simulink model "sampleModel2049_1_sub_sub"  (R2023a)
settings: Solver=VariableStepAuto  StartTime=0.0  StopTime=10.0  RelTol=1e-3
libraries: hdlsllib x3, simulink x2
settings Model: Creator=user1  LastModifiedBy=user1

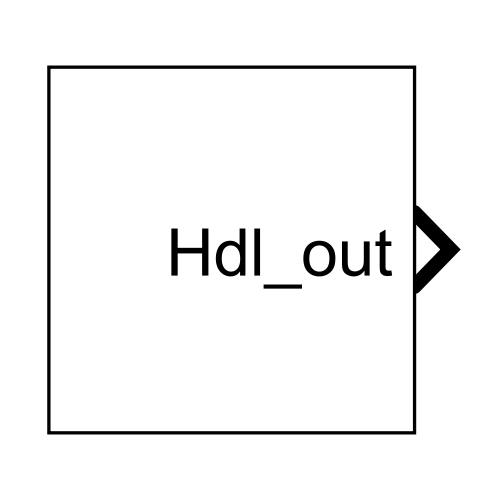
[thumbnail: Simulink's stored preview of the top-level diagram]
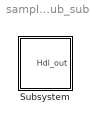
== system sampleModel2049_1_sub_sub ==
  Subsystem : Subsystem

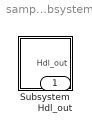
== system sampleModel2049_1_sub_sub/Subsystem ==
  Subsystem : Subsystem
  Hdl_out : Outport  OutDataTypeStr=uint8

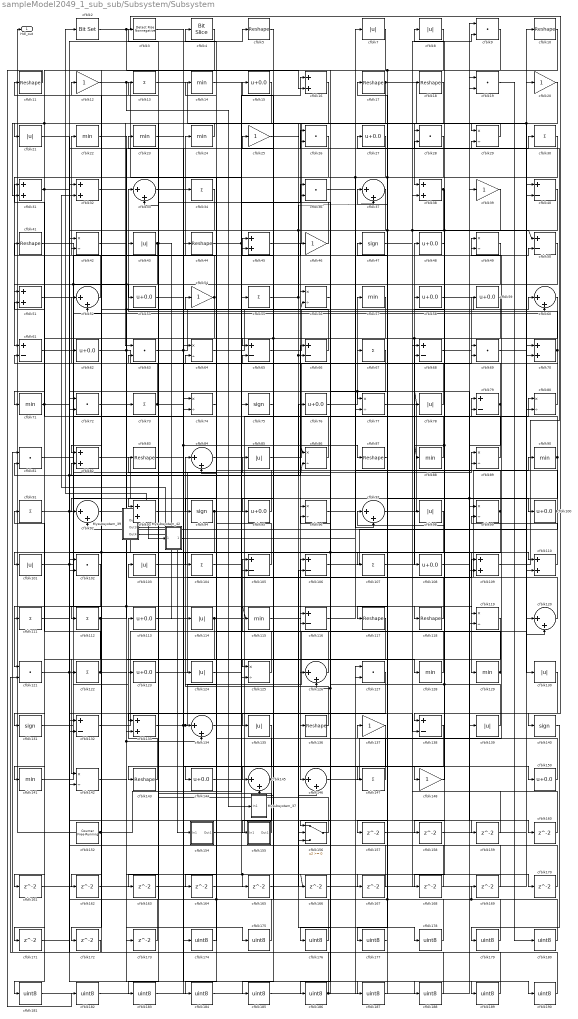
== system sampleModel2049_1_sub_sub/Subsystem/Subsystem ==
  Mysubsystem_37 : Subsystem  TreatAsAtomicUnit=on  RTWFcnName=Mysubsystem_37
      settings: RTWFcnNameOpts=User specified  RTWFileNameOpts=Use function name
  Mysubsystem_39 : Subsystem  TreatAsAtomicUnit=on  RTWFcnName=Mysubsystem_39
      settings: RTWFcnNameOpts=User specified  RTWFileNameOpts=Use function name
  Mysubsystem_42 : Subsystem  TreatAsAtomicUnit=on  RTWFcnName=Mysubsystem_42
      settings: RTWFcnNameOpts=User specified  RTWFileNameOpts=Use function name
  cfblk{5,10..11,17..18,41,44,83,87,117..118,136,143} (13 alike) : Reshape
  cfblk{15,27,48,53,58..59,62,76,95,100,108,113,123,144,150} (15 alike) : Bias  Bias=0.0  SaturateOnIntegerOverflow=off
  cfblk{7..8,21,43,78,85,98,101,103,114,124,130,135,139} (14 alike) : Abs  OutDataTypeStr=uint8  SaturateOnIntegerOverflow=off
  cfblk{9,19,26,28,36,63,69,72,81,102,121,127} (12 alike) : DotProduct  OutDataTypeStr=uint8
  cfblk{13,30,34,55,67,73,91,104,107,111..112,122,147} (13 alike) : Sum  Inputs=+  OutDataTypeStr=uint8
  cfblk{40,50,61,65..66,68,79,105..106,116,132,138} (12 alike) : Sum  Inputs=+-  OutDataTypeStr=uint8
  cfblk{16,31..32,38,45,51,70,82,93,109..110,133} (12 alike) : Sum  OutDataTypeStr=uint8
  cfblk{14,22..24,57,71,88,90,115,128..129,141} (12 alike) : MinMax  OutDataTypeStr=uint8
  cfblk{29,42,49,56,64,74,77,80,86,89,96,99,119,125,142} (15 alike) : Product  Inputs=*/  OutDataTypeStr=uint8  RndMeth=Zero  SaturateOnIntegerOverflow=on
  cfblk{12,20,25,39,46,54,137,148} (8 alike) : Gain  OutDataTypeStr=uint8
  cfblk{33,37,52,60,84,92,97,120,126,134,145..146} (12 alike) : Sum  Inputs=|++  OutDataTypeStr=uint8
  cfblk{47,75,94,131,140} (5 alike) : Signum
  cfblk152 : hdlsllib/Sources/Counter Free-Running  NumBits=16  tsamp=-1
  cfblk154 : Subsystem
      settings: LibrarySourceBlock=|
      | hdlsllib/Ports &
      | Subsystems/Subsystem
  cfblk155 : Subsystem
      settings: LibrarySourceBlock=|
      | hdlsllib/Ports &
      | Subsystems/Subsystem
  cfblk156 : Switch  OutDataTypeStr=uint8  SaturateOnIntegerOverflow=off  InputSameDT=off
  cfblk{157..173} (17 alike) : Delay  SampleTime=1
  cfblk{174..190} (17 alike) : DataTypeConversion  OutDataTypeStr=uint8  SaturateOnIntegerOverflow=off  RndMeth=Floor
  cfblk2 : simulink/Logic and Bit Operations/Bit Set  iBit=0
      settings: LibrarySourceBlock=|
      | hdlsllib/Logic and Bit
      | Operations/Bit Set
  cfblk3 : hdlsllib/Logic and Bit Operations/Detect Rise Nonnegative  vinit=0  OutDataTypeStr=uint8
  cfblk4 : hdlsllib/Logic and Bit Operations/Bit Slice  lidx=7  ridx=0
  Hdl_out : Outport  OutDataTypeStr=uint8
  wires:
  Mysubsystem_42/1(Out1) -> cfblk7/1
  Mysubsystem_39/2(Out2) -> Mysubsystem_42/1(In1)
  Mysubsystem_39/4(Out4) -> cfblk154/1(In1)
  Mysubsystem_39/3(Out3) -> cfblk32/2
  Mysubsystem_39/1(Y) -> cfblk2/1
  cfblk190/1 -> cfblk42/2
  cfblk189/1 -> cfblk42/1
  cfblk83/1 -> cfblk189/1
  cfblk188/1 -> cfblk81/1
  cfblk42/1 -> cfblk188/1
  cfblk187/1 -> cfblk137/1
  cfblk186/1 -> cfblk126/2, cfblk36/2, cfblk32/1
  cfblk185/1 -> cfblk127/2
  cfblk5/1 -> cfblk185/1
  cfblk184/1 -> cfblk127/1
  cfblk49/1 -> cfblk184/1
  cfblk183/1 -> cfblk44/1
  cfblk127/1 -> cfblk183/1
  cfblk182/1 -> cfblk19/2
  cfblk11/1 -> cfblk182/1
  cfblk181/1 -> cfblk19/1
  cfblk180/1 -> cfblk145/2, cfblk17/1, cfblk169/1
  cfblk179/1 -> cfblk25/1
  cfblk140/1 -> cfblk179/1
  cfblk178/1 -> cfblk43/1, cfblk54/1
  cfblk177/1 -> cfblk67/1
  cfblk176/1 -> cfblk72/1
  cfblk67/1 -> cfblk176/1
  cfblk175/1 -> cfblk3/1
  cfblk174/1 -> cfblk124/1
  cfblk3/1 -> cfblk174/1
  cfblk173/1 -> cfblk52/2
  cfblk22/1 -> cfblk173/1
  cfblk172/1 -> cfblk121/2
  cfblk34/1 -> cfblk172/1
  cfblk171/1 -> cfblk132/1
  cfblk170/1 -> cfblk33/2
  cfblk14/1 -> cfblk170/1
  cfblk169/1 -> cfblk63/2
  cfblk168/1 -> cfblk102/1
  cfblk130/1 -> cfblk168/1
  cfblk167/1 -> cfblk105/2
  cfblk166/1 -> cfblk120/2
  cfblk165/1 -> cfblk106/2
  cfblk164/1 -> cfblk146/2
  cfblk163/1 -> cfblk64/1
  cfblk60/1 -> cfblk163/1
  cfblk162/1 -> cfblk38/2
  cfblk37/1 -> cfblk162/1
  cfblk161/1 -> cfblk74/1
  cfblk57/1 -> cfblk161/1
  cfblk160/1 -> cfblk68/1
  cfblk108/1 -> cfblk160/1
  cfblk159/1 -> cfblk99/1
  cfblk158/1 -> cfblk70/1
  cfblk157/1 -> cfblk40/1
  cfblk87/1 -> cfblk157/1
  cfblk104/1 -> cfblk16/1
  cfblk64/1 -> cfblk40/2
  cfblk4/1 -> cfblk21/1
  cfblk16/1 -> cfblk156/2, cfblk66/2
  cfblk120/1 -> cfblk13/1
  cfblk98/1 -> cfblk122/1, cfblk171/1
  cfblk77/1 -> cfblk79/2
  cfblk9/1 -> cfblk156/1
  cfblk56/1 -> cfblk126/1
  cfblk122/1 -> cfblk91/1, cfblk175/1
  cfblk103/1 -> cfblk76/1
  cfblk156/1 -> cfblk23/1
  cfblk94/1 -> cfblk50/2, cfblk111/1
  cfblk10/1 -> cfblk82/1, cfblk177/1
  cfblk142/1 -> cfblk165/1, cfblk166/1
  cfblk105/1 -> cfblk64/2
  cfblk106/1 -> cfblk20/1
  cfblk12/1 -> Mysubsystem_37/1(In1), cfblk55/1
  cfblk73/1 -> cfblk86/1, cfblk125/2, cfblk31/1
  cfblk93/1 -> cfblk66/1
  cfblk69/1 -> cfblk130/1
  cfblk80/1 -> cfblk28/2
  cfblk65/1 -> cfblk9/1
  cfblk72/1 -> cfblk134/2, cfblk187/1
  cfblk55/1 -> cfblk118/1, cfblk37/2
  cfblk85/1 -> cfblk69/1
  cfblk131/1 -> cfblk123/1
  cfblk144/1 -> cfblk106/1
  cfblk68/1 -> cfblk59/1
  cfblk113/1 -> cfblk109/1
  cfblk19/1 -> cfblk180/1
  cfblk112/1 -> cfblk29/2, cfblk115/1, cfblk142/2
  cfblk134/1 -> cfblk75/1
  cfblk63/1 -> cfblk10/1, cfblk110/2
  cfblk119/1 -> cfblk142/1
  cfblk88/1 -> cfblk51/2
  cfblk129/1 -> cfblk96/2, cfblk49/2
  cfblk62/1 -> cfblk56/2, cfblk26/1, cfblk69/2
  cfblk118/1 -> cfblk37/1
  cfblk48/1 -> cfblk138/1
  cfblk132/1 -> cfblk18/1
  cfblk116/1 -> cfblk89/2
  cfblk31/1 -> cfblk77/1, cfblk78/1, cfblk51/1
  cfblk110/1 -> cfblk99/2
  cfblk90/1 -> cfblk107/1, cfblk109/2, cfblk68/2
  cfblk44/1 -> cfblk36/1, cfblk167/1
  cfblk20/1 -> cfblk70/2, cfblk65/1
  cfblk79/1 -> cfblk8/1, cfblk119/2
  cfblk36/1 -> cfblk97/2
  cfblk117/1 -> cfblk131/1
  cfblk95/1 -> cfblk41/1
  cfblk115/1 -> cfblk116/2
  cfblk32/1 -> cfblk125/1
  cfblk53/1 -> cfblk150/1
  cfblk21/1 -> cfblk110/1
  cfblk111/1 -> cfblk119/1
  cfblk75/1 -> cfblk95/1
  cfblk138/1 -> cfblk143/1
  cfblk7/1 -> cfblk112/1
  cfblk17/1 -> cfblk120/1, cfblk53/1
  cfblk50/1 -> cfblk101/1
  cfblk147/1 -> cfblk81/2
  cfblk43/1 -> cfblk72/2, cfblk133/2, cfblk114/1, cfblk93/1
  cfblk124/1 -> cfblk45/2
  cfblk27/1 -> cfblk71/1
  cfblk121/1 -> cfblk86/2, cfblk26/2, cfblk159/1
  cfblk29/1 -> cfblk28/1
  cfblk126/1 -> cfblk84/2
  cfblk78/1 -> cfblk52/1
  cfblk89/1 -> cfblk47/1
  cfblk30/1 -> cfblk92/1, cfblk147/1
  cfblk25/1 -> cfblk178/1
  cfblk46/1 -> cfblk12/1
  cfblk91/1 -> cfblk34/1, cfblk138/2
  cfblk86/1 -> cfblk15/1
  cfblk102/1 -> cfblk121/1
  cfblk133/1 -> cfblk80/2, cfblk134/1, cfblk30/1
  cfblk152/1 -> cfblk49/1, Hdl_out/1
  cfblk145/1 -> cfblk155/1(In1), cfblk61/2
  cfblk28/1 -> cfblk77/2, cfblk164/1
  cfblk47/1 -> cfblk50/1, cfblk9/2
  cfblk84/1 -> cfblk87/1
  cfblk99/1 -> cfblk136/1, cfblk132/2, cfblk62/1
  cfblk76/1 -> cfblk57/1
  cfblk135/1 -> cfblk145/1
  cfblk92/1 -> cfblk129/1
  cfblk150/1 -> cfblk83/1
  cfblk100/1 -> cfblk14/1, cfblk92/2
  cfblk8/1 -> cfblk56/1
  cfblk71/1 -> cfblk5/1, cfblk141/1
  cfblk123/1 -> cfblk89/1
  cfblk38/1 -> cfblk102/2, cfblk158/1
  cfblk148/1 -> cfblk58/1
  cfblk18/1 -> cfblk38/1
  cfblk82/1 -> cfblk96/1
  cfblk40/1 -> cfblk88/1, cfblk148/1, cfblk144/1, cfblk156/3
  cfblk96/1 -> cfblk98/1
  cfblk59/1 -> cfblk135/1, cfblk94/1, cfblk108/1
  cfblk137/1 -> cfblk186/1
  cfblk128/1 -> cfblk45/1
  cfblk136/1 -> cfblk84/1
  cfblk66/1 -> cfblk11/1
  cfblk52/1 -> cfblk22/1
  cfblk114/1 -> cfblk39/1, cfblk133/1
  cfblk39/1 -> cfblk117/1, cfblk104/1
  cfblk33/1 -> cfblk74/2
  cfblk155/1(Out1) -> cfblk103/1
  cfblk41/1 -> cfblk139/1, cfblk73/1
  cfblk141/1 -> cfblk85/1
  cfblk61/1 -> cfblk116/1
  cfblk51/1 -> cfblk100/1
  cfblk2/1 -> cfblk140/1, cfblk16/2
  cfblk125/1 -> cfblk105/1
  cfblk81/1 -> cfblk60/2
  cfblk143/1 -> cfblk113/1
  cfblk101/1 -> cfblk46/1, cfblk190/1
  cfblk13/1 -> cfblk146/1
  cfblk26/1 -> cfblk61/1
  cfblk97/1 -> cfblk79/1
  cfblk45/1 -> cfblk29/1
  cfblk15/1 -> cfblk31/2, cfblk181/1
  cfblk107/1 -> cfblk48/1
  cfblk74/1 -> cfblk4/1
  cfblk58/1 -> cfblk60/1
  cfblk24/1 -> cfblk63/1
  cfblk146/1 -> cfblk90/1
  cfblk139/1 -> cfblk97/1, cfblk82/2
  cfblk109/1 -> cfblk27/1
  cfblk23/1 -> cfblk128/1
  cfblk70/1 -> cfblk33/1, cfblk65/2
  cfblk54/1 -> cfblk24/1, cfblk93/2
  cfblk154/1(Out1) -> cfblk80/1

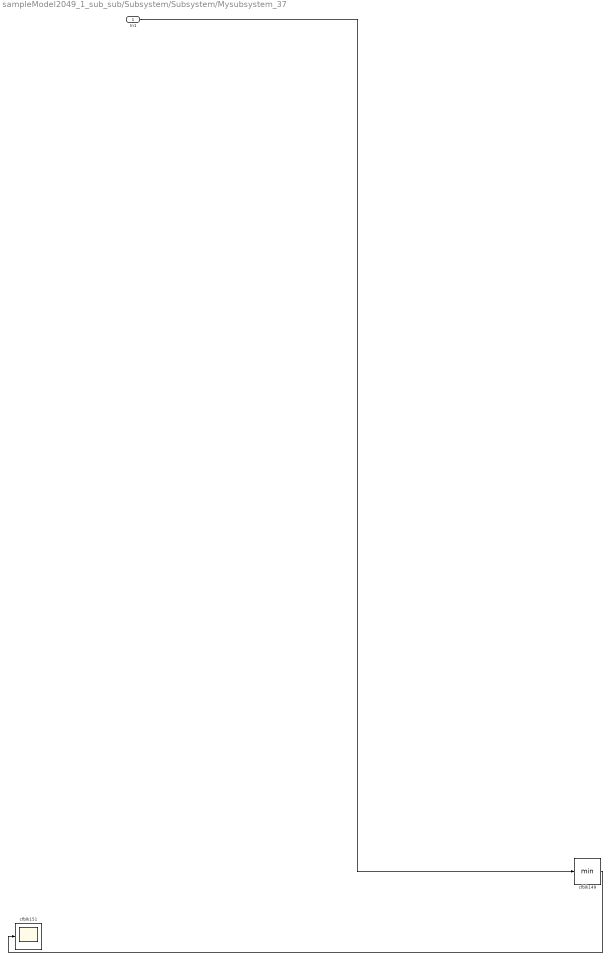
== system sampleModel2049_1_sub_sub/Subsystem/Subsystem/Mysubsystem_37 ==
  In1 : Inport
  cfblk149 : MinMax
  cfblk151 : Scope
  wires:
  In1/1 -> cfblk149/1
  cfblk149/1 -> cfblk151/1

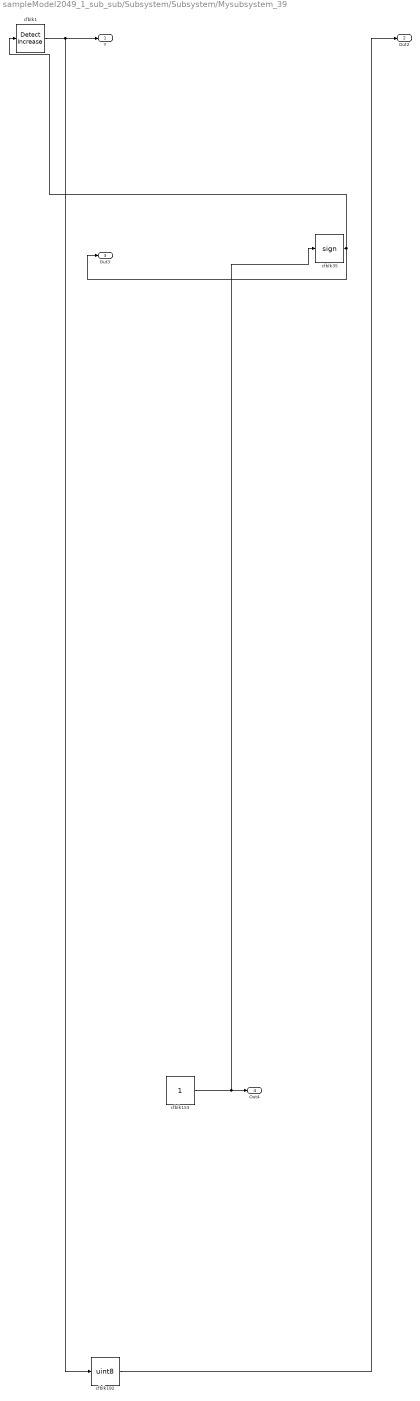
== system sampleModel2049_1_sub_sub/Subsystem/Subsystem/Mysubsystem_39 ==
  cfblk1 : simulink/Logic and Bit Operations/Detect Increase  vinit=0.0  OutDataTypeStr=boolean
      settings: LibrarySourceBlock=|
      | hdlsllib/Logic and Bit
      | Operations/Detect
      | Increase
  cfblk153 : Constant  SampleTime=-1
  cfblk192 : DataTypeConversion  OutDataTypeStr=uint8  SaturateOnIntegerOverflow=off  RndMeth=Floor
  cfblk35 : Signum
  Y : Outport
  Out2 : Outport  Port=2
  Out3 : Outport  Port=3
  Out4 : Outport  Port=4
  wires:
  cfblk35/1 -> Out3/1, cfblk1/1
  cfblk153/1 -> Out4/1, cfblk35/1
  cfblk1/1 -> Y/1, cfblk192/1
  cfblk192/1 -> Out2/1

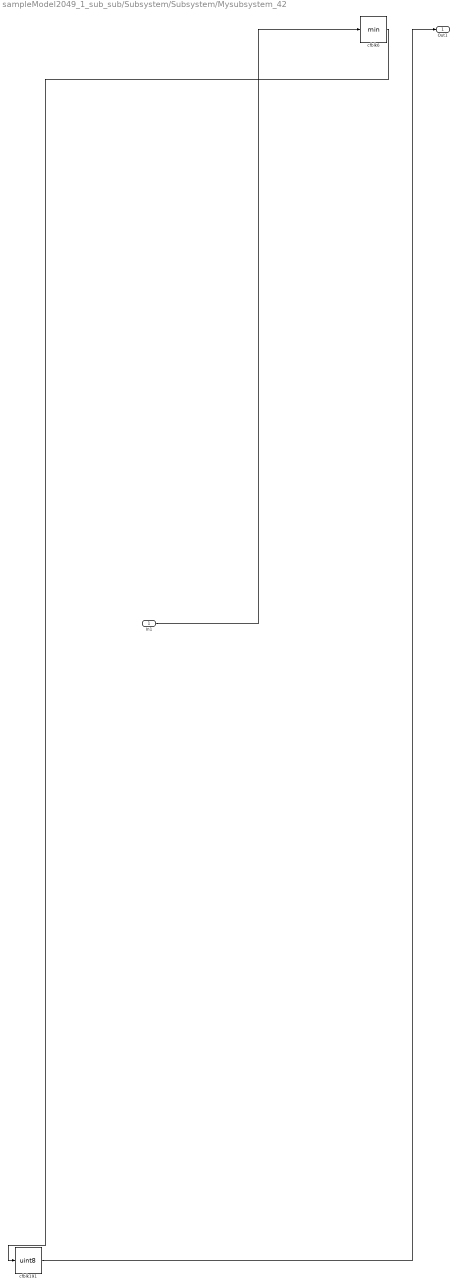
== system sampleModel2049_1_sub_sub/Subsystem/Subsystem/Mysubsystem_42 ==
  In1 : Inport
  cfblk191 : DataTypeConversion  OutDataTypeStr=uint8  SaturateOnIntegerOverflow=off  RndMeth=Floor
  cfblk6 : MinMax
  Out1 : Outport
  wires:
  cfblk6/1 -> cfblk191/1
  cfblk191/1 -> Out1/1
  In1/1 -> cfblk6/1

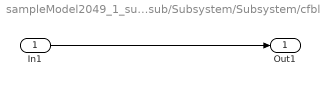
== system sampleModel2049_1_sub_sub/Subsystem/Subsystem/cfblk154 ==
  In1 : Inport
  Out1 : Outport
  wires:
  In1/1 -> Out1/1

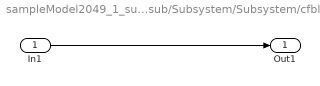
== system sampleModel2049_1_sub_sub/Subsystem/Subsystem/cfblk155 ==
  In1 : Inport
  Out1 : Outport
  wires:
  In1/1 -> Out1/1
